simulink model "skid_steer_model"  (R2015a)
settings: Solver=ode3  StartTime=0.0  StopTime=50  RelTol=1e-3
values from neighbouring files (symbols this model uses):
  Ts = 60e-3    (= 0.06)    [Diseno_controlador_LQR_skid_steer.m]
settings Model: CovModelRefEnable=off  Creator=haroldfmurcia  LastModifiedBy=haroldfmurcia
settings DataIOCC: SaveFormat=Dataset
settings HardwareCC: ProdBitPerPointer=64  ProdLargestAtomicFloat=Float  ProdIntDivRoundTo=Zero  ProdEndianess=LittleEndian  ProdHWDeviceType=Specified
settings GRTTargetCC: GeneratePreprocessorConditionals=Use local settings

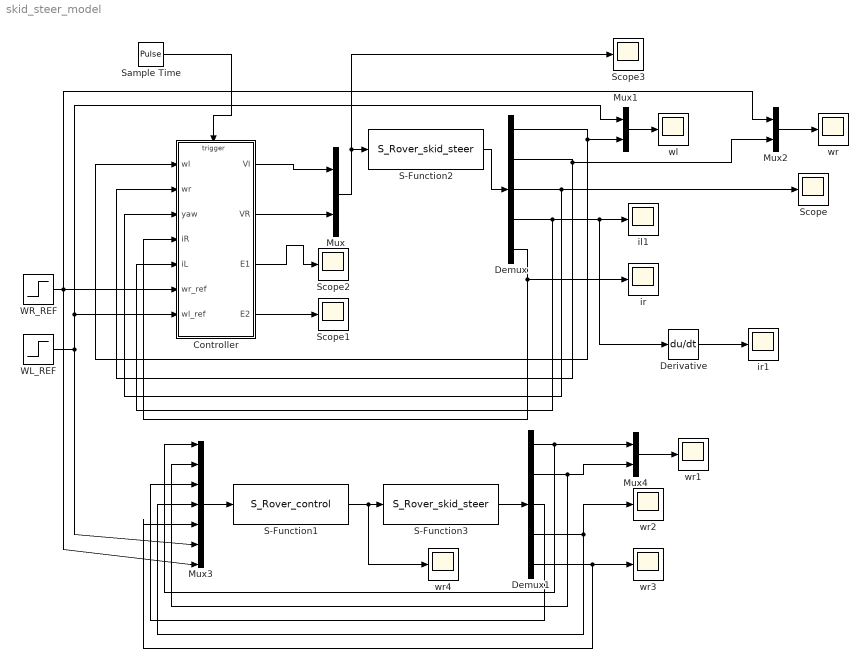
== system skid_steer_model ==
  Controller : Subsystem
  Demux : Demux  Outputs=5
  Demux1 : Demux  Outputs=5
  Derivative : Derivative
  Mux{,1..2,4} (4 alike) : Mux  Inputs=2
  Mux3 : Mux  Inputs=7
  S-Function1 : S-Function  FunctionName=S_Rover_control  SFunctionDeploymentMode=off  EnableBusSupport=off
  S-Function2 : S-Function  FunctionName=S_Rover_skid_steer  SFunctionDeploymentMode=off  EnableBusSupport=off
  S-Function3 : S-Function  FunctionName=S_Rover_skid_steer  SFunctionDeploymentMode=off  EnableBusSupport=off
  Sample Time : DiscretePulseGenerator  PulseType=Time based  Period=Ts  PulseWidth=10  SampleTime=1e-3
  Scope{,1..3} (4 alike) : Scope
      Scope settings: TimeRange=auto  MaxDataPoints=5000  SaveToWorkspace=off  SaveName=ScopeData  YMin=-0.61679  YMax=5.54233  SampleTime=-1
      Scope1 settings: TimeRange=auto  MaxDataPoints=5000  SaveToWorkspace=off  SaveName=ScopeData4  YMin=-1.25  YMax=1.25  SampleTime=-1
      Scope2 settings: TimeRange=auto  MaxDataPoints=5000  SaveToWorkspace=off  SaveName=ScopeData8  YMin=-3.84725  YMax=8.70895  SampleTime=-1
      Scope3 settings: TimeRange=auto  MaxDataPoints=5000  SaveToWorkspace=off  SaveName=ScopeData3  YMin=-124.70891  YMax=124.96766  SampleTime=-1
  WL_REF : Step  Time=5  Before=1  After=0.5  SampleTime=0
  WR_REF : Step  Time=30  Before=1  After=1.5  SampleTime=0
  il1 : Scope
      settings: TimeRange=auto  MaxDataPoints=5000  SaveToWorkspace=off  SaveName=ScopeData5  YMin=-6.35578  YMax=23.2116  SampleTime=-1
  ir : Scope
      settings: TimeRange=auto  MaxDataPoints=5000  SaveToWorkspace=off  SaveName=ScopeData6  YMin=-6.8481  YMax=37.14237  SampleTime=-1
  ir1 : Scope
      settings: TimeRange=auto  MaxDataPoints=5000  SaveToWorkspace=off  SaveName=ScopeData7  YMin=-34.07938  YMax=41.49955  SampleTime=-1
  wl : Scope
      settings: TimeRange=auto  MaxDataPoints=5000  SaveToWorkspace=off  YMin=-0.20599  YMax=1.63682  SampleTime=-1
  wr{,1..4} (5 alike) : Scope
      wr settings: TimeRange=auto  MaxDataPoints=5000  SaveToWorkspace=off  SaveName=ScopeData2  YMin=-0.271  YMax=1.89419  SampleTime=-1
      wr1 settings: TimeRange=auto  MaxDataPoints=5000  SaveToWorkspace=off  SaveName=ScopeData9  YMin=-0.25547  YMax=1.77331  SampleTime=-1
      wr2 settings: TimeRange=auto  MaxDataPoints=5000  SaveToWorkspace=off  SaveName=ScopeData10  YMin=-45.38843  YMax=19.47524  SampleTime=-1
      wr3 settings: TimeRange=auto  MaxDataPoints=5000  SaveToWorkspace=off  SaveName=ScopeData11  YMin=-15.77008  YMax=38.5341  SampleTime=-1
      wr4 settings: TimeRange=auto  MaxDataPoints=5000  SaveToWorkspace=off  SaveName=ScopeData12  YMin=-125.00000  YMax=125.00000  SampleTime=-1
  wires:
  Demux/3 -> Controller/3(yaw), Scope/1
  Demux/2 -> Mux2/2, Controller/2(wr)
  Demux/1 -> Mux1/2, Controller/1(wl)
  Sample Time/1 -> Controller/Trigger
  Demux/4 -> Derivative/1, il1/1, Controller/5(iL)
  Demux/5 -> Controller/4(iR), ir/1
  Controller/1(Vl) -> Mux/1
  Controller/2(VR) -> Mux/2
  Controller/4(E2) -> Scope1/1
  Controller/3(E1) -> Scope2/1
  WR_REF/1 -> Mux3/7, Mux2/1, Controller/6(wr_ref)
  WL_REF/1 -> Controller/7(wl_ref), Mux1/1, Mux3/6
  Mux1/1 -> wl/1
  Mux2/1 -> wr/1
  Derivative/1 -> ir1/1
  S-Function2/1 -> Demux/1
  Mux/1 -> S-Function2/1, Scope3/1
  Mux3/1 -> S-Function1/1
  S-Function1/1 -> wr4/1, S-Function3/1
  S-Function3/1 -> Demux1/1
  Mux4/1 -> wr1/1
  Demux1/1 -> Mux3/1, Mux4/1
  Demux1/2 -> Mux3/2, Mux4/2
  Demux1/4 -> wr2/1, Mux3/4
  Demux1/5 -> Mux3/5, wr3/1
  Demux1/3 -> Mux3/3

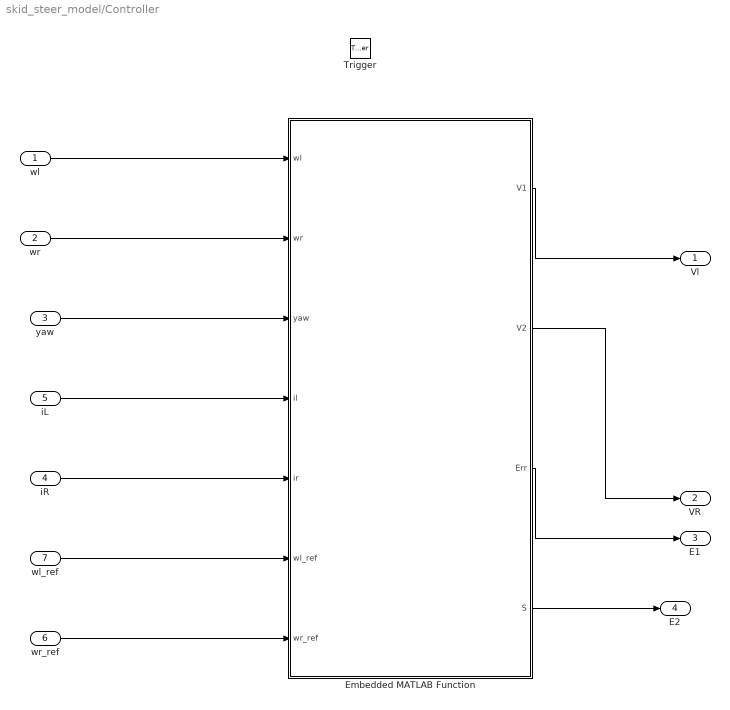
== system skid_steer_model/Controller ==
  wl : Inport
  wr : Inport  Port=2
  yaw : Inport  Port=3
  iR : Inport  Port=4
  iL : Inport  Port=5
  wr_ref : Inport  Port=6
  wl_ref : Inport  Port=7
  Trigger : TriggerPort
  Embedded MATLAB Function : MATLAB Function  TreatAsAtomicUnit=on
      settings: PermitHierarchicalResolution=ParametersOnly
  Vl : Outport
  VR : Outport  Port=2
  E1 : Outport  Port=3
  E2 : Outport  Port=4
  wires:
  Embedded MATLAB Function/1(V1) -> Vl/1
  wl/1 -> Embedded MATLAB Function/1(wl)
  wr/1 -> Embedded MATLAB Function/2(wr)
  Embedded MATLAB Function/2(V2) -> VR/1
  yaw/1 -> Embedded MATLAB Function/3(yaw)
  Embedded MATLAB Function/3(Err) -> E1/1
  Embedded MATLAB Function/4(S) -> E2/1
  wl_ref/1 -> Embedded MATLAB Function/6(wl_ref)
  wr_ref/1 -> Embedded MATLAB Function/7(wr_ref)
  iR/1 -> Embedded MATLAB Function/5(ir)
  iL/1 -> Embedded MATLAB Function/4(il)

== matlab function skid_steer_model/Controller/Embedded MATLAB Function ==
  data: wl input; V1 output; wr input; V2 output; yaw input; il input; ir input; Err output; S output; wl_ref input; wr_ref input
function [V1,V2,Err,S]  = fcn(wl,wr,yaw,il,ir,wl_ref,wr_ref)

ref_wl=wl_ref;
ref_wr=wr_ref;
ref_il=-40;
ref_ir=-40;
ref_theta=pi;

Ts=60e-3;

Kp=2.7;
Ti=.6;
Td=0.15*0;

persistent Ui_1_wl Ui_1_wr error_1_wl error_1_wr U_wr_1 U_wl_1 il_1 ir_1 wl_1 wr_1 wr_ref_1 wl_ref_1 il_ref_1;

if isempty(il_ref_1); il_ref_1=0;   end;
if isempty(wl_ref_1); wl_ref_1=0;   end;
if isempty(wr_ref_1); wr_ref_1=0;   end;
if isempty(wl_1); wl_1=0;   end;
if isempty(wr_1); wr_1=0;   end;
if isempty(il_1); il_1=0;   end;
if isempty(ir_1); ir_1=0;   end;

if isempty(U_wl_1); U_wl_1=0;   end;
if isempty(U_wr_1); U_wr_1=0;   end;
if isempty(Ui_1_wl); Ui_1_wl=0;   end;
if isempty(Ui_1_wr); Ui_1_wr=0;   end;
if isempty(error_1_wl); error_1_wl=0;   end;
if isempty(error_1_wr); error_1_wr=0;   end;                                                                                                                                


%% MODELO
w_l=wl;
w_r=wr;
theta=yaw;
I_l=il;
I_r=ir;

N=16;
r=0.2;
L=0.61/2;  %ancho del carro
a=0.62/2;  %Largo del carro
m=58;
Kpwm=0.1237;
g=9.81;
Yr=0.45;
Yl=Yr;
Kbr=0.0592;
Kbl=0.0637;
Kmr=0.0946;
Kml=0.0770;
Xg=-0.079; 
La= 0.081;
Ra=0.33;
I=15;
u_r=0.001;
u_l=0.8;

%

P=1/(Yl+Yr)*[Yr Yl;-1 1];
q_dot=P*[w_l;w_r];
x_dot=q_dot(1);
w_rover=q_dot(2);
y_dot=w_rover*Xg;

x1r_dot=x_dot-L*w_rover;
x2r_dot=x_dot+L*w_rover;
y1r_dot=y_dot+a*w_rover;
y3r_dot=y_dot-a*w_rover;
Rx=u_r*m*g/2*(sign(x1r_dot)+sign(x2r_dot));
Fy=u_l*m*g/2*(sign(y1r_dot)+sign(y3r_dot));
Mr=u_l*a*m*g/2*(sign(y1r_dot)-sign(y3r_dot))+u_r*L*m*g/2*(sign(x2r_dot)-sign(x1r_dot));


M_b=[m 0;...
     0 m*Xg^2+I];

C_b=m*Xg*w_rover*[0 1;-1 0];
R_b=[Rx*cos(theta)-Fy*sin(theta);...
     Xg*(Rx*sin(theta)+Fy*cos(theta))+Mr];
 
B_b=1/r*[1 1;-L L];

Km=N*[Kml 0;0 Kmr];

%% Dynamic matrix %%%%%%%%%%%%%%%%%%%%%%%%%%%%%%

Ac=[-inv(M_b*P)*C_b*P zeros(2,1) inv(M_b*P)*B_b*Km;...
    -1/(Yl+Yr) 1/(Yl+Yr) zeros(1,3);...
    -Kbl*N/La 0 0 -Ra/La 0;...
    0 -Kbr*N/La 0 0 -Ra/La];

Bc=[zeros(3,2);Kpwm/La 0;0 Kpwm/La];




Cc=eye(5);

Dc=0;


eml.extrinsic('ss');
eml.extrinsic('c2d');
eml.extrinsic('ssdata');

eml.extrinsic('matrix.h');

%G=ss(Ac,Bc,Cc,Dc);
%Gd=c2d(G,Ts);
%[Ad,Bd,Cd,Dd,TT]=ssdata(Gd);

A=[ 0.9401    0.0548         0    0.0093    0.0039;
    0.0549    0.9396         0    0.0032    0.0115;
   -0.0126    0.0126    1.0000   -0.0000    0.0001;
   -0.6489   -0.0196         0    0.7797   -0.0014;
   -0.0183   -0.6030         0   -0.0011    0.7793];


B=[ 0.0004    0.0002;
    0.0002    0.0006;
   -0.0000    0.0000;
    0.0812   -0.0000;
   -0.0000    0.0812];

Cd=[         0         0    1.0000         0         0;
    0.1000    0.1000         0         0         0];

Dd=zeros(2,2);



F=[inv(M_b*P)*R_b;zeros(3,1)];

%% Errores

error_wr=ref_wr-wr;
error_wl=ref_wl-wl;
error_il=20-il;
error_ir=20-ir;
error_theta=ref_theta-yaw;

%% Saturaciones

E2=error_wr;
if(E2)>0
    S2=1;
else
    S2=-1;
end


E1=error_wl;
if(E1)>1
    S1=1;
elseif (E1)<-1
    S1=-1;
else
    S1=E1;
end



E3=error_theta;
if(E3)>1
    S3=1;
elseif(E3)<-1
    S3=-1;
else
    S3=E3;
end


E4=error_il;
if(E4)>1
    S4=1;
elseif(E4)<-1
    S4=-1;
else
    S4=E4;
end

E5=error_ir;
if(E5)>1
    S5=1;
elseif(E5)<-1
     S5=-1;
else
    S5=E5;
end




%% Wl

Up_wl=Kp*error_wl;
Ui_wl = Kp*Ts/(Ti)*error_1_wl+Ui_1_wl;
Ud_wl = Kp*Td/(Ts)*(error_wl-error_1_wl);
U_wl= (Up_wl +Ui_wl + Ud_wl )*100/12; ;


%% Wr

Up_wr=Kp*error_wr;
Ui_wr = Kp*Ts/(Ti)*error_1_wr+Ui_1_wr;
Ud_wr = Kp*Td/(Ts)*(error_wr-error_1_wr);
U_wr=( Up_wr + Ui_wr+ Ud_wr)  *100/12; 


%%
K1=5;
q1=20;

K6=-100;
q6=1;
ir_dot=(ir-ir_1)/Ts;
il_dot=(il-il_1)/Ts;
wl_dot=(wl-wl_1)/Ts;
wr_dot=(wr-wr_1)/Ts;
wr_ref_dot=(wr_ref-wr_ref_1)/Ts;
wl_ref_dot=(wl_ref-wl_ref_1)/Ts;



%il_ref= ( (wl_ref_dot -K1*E1 -q1*S1 -A(1,1)*wl-A(1,2)*wr-A(1,5)*ir)/A(1,4) );


%il_ref_dot=(il_ref-il_ref_1)/Ts;

%U_wl= (il_ref_dot-K6*E6 -q6*S6 -A(4,1)*wl-A(4,4)*il)/B(4,1);

ir_1=ir;
il_1=il;
wl_1=wl;
wr_1=wr;
wr_ref_1=wr_ref;
wl_ref_1=wl_ref;

%U_wl= ( ( A(4,4)/(A(1,4)-A(2,4)*A(1,5)/A(2,5)) ) *( 0*wl_ref_dot +K1*error_wl +q1*S1 -A(1,1)*wl-A(1,2)*wr-A(1,5)/A(2,5)*(wr_dot)-A(2,1)*wl-A(2,2)*wr ) -il_dot+A(4,1)*wl )/-B(4,1);
%U_wl= (il_ref_dot-K5*E5 -q5*S5 -A(4,1)*wl-A(4,4)*il)/B(4,1);
%U_wr= ( ( A(5,5)/(A(2,5)-A(2,4)*A(1,5)/A(1,4)) ) *(0* wr_ref_dot +K1*error_wr +q1*S2 -A(2,1)*wl-A(2,2)*wr-A(2,4)/A(1,4)*(wl_dot)-A(1,1)*wl-A(1,2)*wr ) -ir_dot+A(5,2)*wr )/-B(5,2);

R_dot=[wl_ref_dot;wr_ref_dot;0;0;0];
Err=[E1;E2;E3;E4;E5];
S=[S1;S2;S3;S4;S5];
x=[wl;wr;yaw;il;ir];
C=[0 0 0 1 0;0 0 0 0 1];
Uc=inv(C*B)*C*(R_dot-A*x +q1*S+K1*Err )
%U_wl=Uc(1);
%U_wr=Uc(2);


U_wl_1=U_wl;
U_wr_1=U_wr;
%%

if ( U_wl >  100 ) U_wl = 100; end
if ( U_wl < -100 ) U_wl = -100; end

if ( U_wr >  100 ) U_wr = 100; end
if ( U_wr < -100 ) U_wr = -100; end

%Ui_wl=U_wl-Up_wl-Ud_wl; %Anti Reset-Windup
%Ui_wr=U_wr-Up_wr-Ud_wr; %Anti Reset-Windup

error_1_wl = error_wl;
Ui_1_wl =Ui_wl;

error_1_wr = error_wr;
Ui_1_wr =Ui_wr;

V1=U_wl;%;*100/12.1;
V2=U_wr;%;*100/12.1;
